simulink model "ukfDebug"  (R2024b)
settings: Solver=VariableStepAuto  StartTime=0.0  StopTime=10.0  RelTol=1e-3
undefined symbols (not defined in the file or in its folder): Aero, Motor, Uav
libraries: sharedTrackingLibrary x1
settings Model: Creator=jski306  LastModifiedBy=jski306

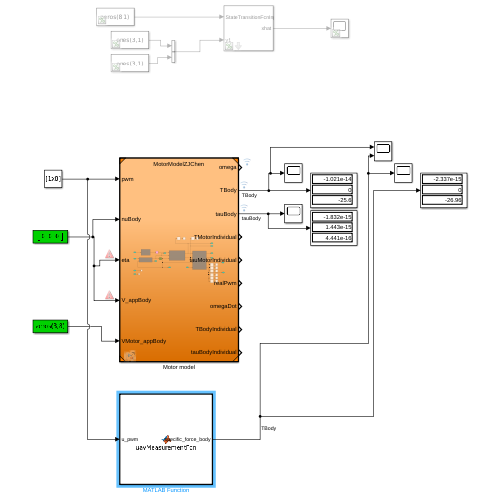
[thumbnail: Simulink's stored preview of the top-level diagram]
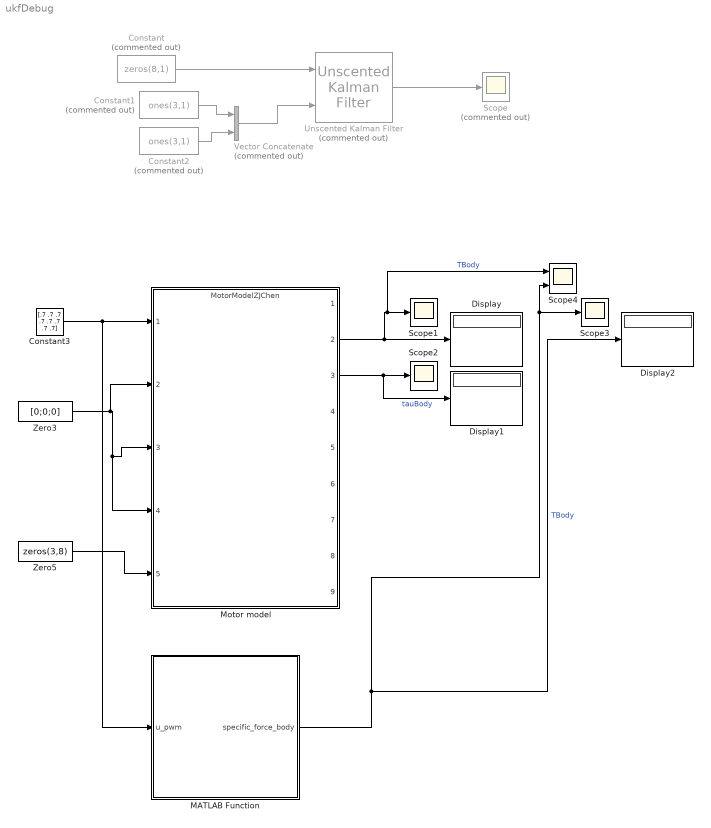
== system ukfDebug ==
  Constant : Constant  Commented=on  Value=zeros(8,1)
  Constant1 : Constant  Commented=on  Value=ones(3,1)
  Constant2 : Constant  Commented=on  Value=ones(3,1)
  Constant3 : Constant  Value=[.7 .7 .7 .7 .7 .7 .7 .7]
  Display : Display
  Display1 : Display
  Display2 : Display
  MATLAB Function : MATLAB Function  TreatAsAtomicUnit=on
  Motor model : ModelReference  ModelNameDialog=MotorModelZJChen  SimulationMode=Normal  ModelReferenceVersion=13.7
  Scope : Scope  Commented=on
  Scope1 : Scope
  Scope2 : Scope
  Scope3 : Scope
  Scope4 : Scope  NumInputPorts=2
  Unscented Kalman Filter : sharedTrackingLibrary/Unscented Kalman Filter  Commented=on  StateTransitionFcn=uavStateFcn  HasAdditiveProcessNoise=Additive  ProcessNoise=UKF_full.ProcessNoise  HasTimeVaryingProcessNoise=off  HasStateTransitionFcnExtraArgument=1  InitialState=UKF_full.InitialState  InitialStateCovariance=UKF_full.InitialCovariance  Alpha=UKF_full.Alpha  Beta=UKF_full.Beta  Kappa=UKF_full.Kappa  MeasurementFcn1=uavMeasurementFcn  HasMeasurementEnablePort1=off  HasAdditiveMeasurementNoise1=Additive  MeasurementNoise1=UKF_full.MeasurementNoise  HasTimeVaryingMeasurementNoise1=off  HasMeasurementFcnExtraArgument1=0  HasMeasurementWrapping1=off  MeasurementFcn2=myMeasurementFcn  HasMeasurementEnablePort2=off  HasAdditiveMeasurementNoise2=Additive  MeasurementNoise2=1  HasTimeVaryingMeasurementNoise2=off  HasMeasurementFcnExtraArgument2=0  HasMeasurementWrapping2=off  MeasurementFcn3=myMeasurementFcn  HasMeasurementEnablePort3=off  HasAdditiveMeasurementNoise3=Additive  MeasurementNoise3=1  HasTimeVaryingMeasurementNoise3=off  HasMeasurementFcnExtraArgument3=0  HasMeasurementWrapping3=off  MeasurementFcn4=myMeasurementFcn  HasMeasurementEnablePort4=off  HasAdditiveMeasurementNoise4=Additive  MeasurementNoise4=1  HasTimeVaryingMeasurementNoise4=off  HasMeasurementFcnExtraArgument4=0  HasMeasurementWrapping4=off  MeasurementFcn5=myMeasurementFcn  HasMeasurementEnablePort5=off  HasAdditiveMeasurementNoise5=Additive  MeasurementNoise5=1  HasTimeVaryingMeasurementNoise5=off  HasMeasurementFcnExtraArgument5=0  HasMeasurementWrapping5=off  EnableMultirate=off  StateTransitionFcnSampleTime=1  MeasurementFcn1SampleTime=1  MeasurementFcn2SampleTime=1  MeasurementFcn3SampleTime=1  MeasurementFcn4SampleTime=1  MeasurementFcn5SampleTime=1  UseCurrentEstimator=on  OutputStateCovariance=off  DataType=double  SampleTime=1  NumberOfMeasurements=1
      settings: LibrarySourceBlock=cstblocks/State Estimation/Unscented Kalman Filter
  Vector Concatenate : Concatenate  Commented=on
  Zero3 : Constant  Value=[0;0;0]  OutDataTypeStr=Inherit: Inherit via back propagation
  Zero5 : Constant  Value=zeros(3,8)  OutDataTypeStr=Inherit: Inherit via back propagation
  wires:
  Unscented Kalman Filter/1 -> Scope/1
  Constant/1 -> Unscented Kalman Filter/1
  Vector Concatenate/1 -> Unscented Kalman Filter/2
  Constant1/1 -> Vector Concatenate/1
  Constant2/1 -> Vector Concatenate/2
  Zero5/1 -> Motor model/5
  Zero3/1 -> Motor model/2, Motor model/3, Motor model/4
  Constant3/1 -> MATLAB Function/1(u_pwm), Motor model/1
  Motor model/2 -> Scope4/1, Scope1/1, Display/1  "TBody"
  Motor model/3 -> Display1/1, Scope2/1  "tauBody"
  MATLAB Function/1(specific_force_body) -> Display2/1, Scope4/2, Scope3/1  "TBody"

== matlab function ukfDebug/MATLAB Function ==
  data: u_pwm input; Motor parameter; Uav parameter; Aero parameter; specific_force_body output
function specific_force_body  = uavMeasurementFcn(u_pwm, Motor, Uav, Aero)
%uavMeasurementFcn Predicts sensor readings by replicating the plant model.
%   This version uses the user-provided QuatToRot function to ensure an
%   exact match with the ground-truth simulation's coordinate transformations.

    % --- 3. Predict Accelerometer Reading --- 
    % a) Calculate the wrench from motors (TBody)
    params.C_tau  = Motor.C_TAU;
    params.Kt     = Motor.K_T;
    params.Ke     = Motor.K_E;
    params.R      = Motor.R;
    params.I0     = Motor.I_0;
    params.V_off  = Motor.Volt_offset;
    params.mv     = Motor.volt_slope;
    mass = 0.95;
    % b) Rebuild the B-matrix
    N_motors = size(u_pwm, 1);
    params.B_matrix = zeros(6, N_motors);
    % d) B-Matrix construction
    kf_vec = 0.5 * Uav.RHO_AIR * Aero.Cz3P.coefs(1) * (Uav.D_PROP.^2) .* Uav.A_PROP;
    km_vec = params.C_tau;

    for m = 1:N_motors
        t_m = [0; 0; -kf_vec(m)];
        tau_m = [0; 0; -Uav.ROTOR_DIRECTION(m) * km_vec(m)];
        R_m_b = Uav.R_MOTOR_TO_BODY(:,:,m);
        T_body_i = R_m_b * t_m;
        tau_body_i = R_m_b * tau_m;

        % Select only the first 3 elements [x,y,z] for the position vector
        r_i = Uav.MotorLoc(m, 1:3)';
        
        tau_from_thrust = cross(r_i, T_body_i);
        params.B_matrix(:, m) = [T_body_i; tau_body_i + tau_from_thrust];
    end

    W_ss = pwm_to_wrench(u_pwm, params);
    TBody = W_ss(1:3);

    % c) Calculate specific force (acceleration from thrust) in the body frame
    specific_force_body = TBody / mass;
end

function R = QuatToRot( q )
%QUATTOROT Convert quaternion to rotation matrix
%   This is the exact function used by the ground-truth sensor.
    W = q(1);
    X = q(2);
    Y = q(3);
    Z = q(4);
    
    xx = X * X;
    xy = X * Y;
    xz = X * Z;
    xw = X * W;
    yy = Y * Y;
    yz = Y * Z;
    yw = Y * W;
    
    zz = Z * Z;
    zw = Z * W;
    m00 = 1 - 2 * ( yy + zz );
    m01 =     2 * ( xy - zw );
    m02 =     2 * ( xz + yw );
    m10 =     2 * ( xy + zw );
    m11 = 1 - 2 * ( xx + zz );
    m12 =     2 * ( yz - xw );
    m20 =     2 * ( xz - yw );
    m21 =     2 * ( yz + xw );
    m22 = 1 - 2 * ( xx + yy );
    
    R = [m00 m01 m02;
         m10 m11 m12;
         m20 m21 m22];   
end



function W_ss = pwm_to_wrench(pwm_inputs, params)
% pwm_to_wrench - Computes the steady-state wrench from individual motor PWM inputs.
%
% Inputs:
%    pwm_inputs - An Nx1 vector of PWM commands (scaled 0 to 1).
%    params     - A structure containing motor and vehicle parameters.
%                 .N         : Number of motors.
%                 .C_tau, .Kt, .Ke, .R, .mv, .V_off, .I0 : Per-motor dynamics params.
%                 .B_matrix  : The 6xN matrix mapping squared rotor speeds to wrench.
%
% Outputs:
%    W_ss - The resulting steady-state wrench vector [Fx; Fy; Fz; Tx; Ty; Tz].

    % --- 1. Calculate Squared Rotor Speeds from PWM ---
    % This helper function is the same as your 'calculate_omega_sq'
    omega_ss_sq = calculate_omega_sq_from_pwm(pwm_inputs, params);
    
    % --- 2. Calculate Final Wrench using the B-Matrix ---
    % The B-matrix maps the contribution of each motor's squared speed to the total wrench.
    W_ss = params.B_matrix * omega_ss_sq;
end

function omega_sq = calculate_omega_sq_from_pwm(u, motor_params)
    % This is your original 'calculate_omega_sq' function, just renamed for clarity.
    % It solves the quadratic equation for motor speed.
    A_quad_vec = motor_params.C_tau(:); Kt_vec = motor_params.Kt(:);
    Ke_vec = motor_params.Ke(:); R_vec = motor_params.R(:);
    mv_vec = motor_params.mv(:); V_off_vec = motor_params.V_off(:);
    I0_vec = motor_params.I0(:);
    
    B_quad_vec = (Kt_vec .* Ke_vec) ./ R_vec;
    C_quad_vec = -(Kt_vec ./ R_vec) .* (mv_vec .* u + V_off_vec - I0_vec .* R_vec);
    
    discriminant = B_quad_vec.^2 - 4 * A_quad_vec .* C_quad_vec;
    discriminant(discriminant < 0) = 0; % Prevent complex results
    
    omega_ss = (-B_quad_vec + sqrt(discriminant)) ./ (2 * A_quad_vec);
    omega_sq = omega_ss.^2;
end
